simulink model "ExampleAdditionalVehicle"  (Simulink 9.2)
settings: Solver=FixedStepDiscrete  StartTime=0.0  StopTime=inf  FixedStep=0.001  RelTol=1e-3  EnableMultiTasking=on
libraries: rFproPhysicsLib x15, simulink x2
settings Model: Creator=enewton  LastModifiedBy=SeanKavanagh  ParamWorkspaceSource=ReferencedWorkspace  TunableVars=LOCAL_PORT_RECV,REMOTE_PORT_RECV,gCGHeight,gFrontTrack,gFrontWheelRadius,gLeftWheelBase,gRearTrack,gRearWheelRadius,gRightWheelBase  TunableVarsStorageClass=Auto,Auto,Auto,Auto,Auto,Auto,Auto,Auto,Auto  TunableVarsTypeQualifier=,,,,,,,,
settings OptimizationCC: DefaultParameterBehavior=Inlined  ExpressionDepthLimit=2147483647
settings DebuggingCC: SolverPrmCheckMsg=warning
settings HardwareCC: TargetBitPerPointer=64  TargetBitPerSizeT=64  TargetBitPerPtrDiffT=64  TargetLongLongMode=on  TargetIntDivRoundTo=Zero  TargetEndianess=LittleEndian  TargetWordSize=64  TargetHWDeviceType=MATLAB Host  ProdEqTarget=off
settings RTWCC: SystemTargetFile=rfpro.tlc  MakeCommand="make_rtw OPTS=\"-DRUN_PHYSICS\""  TemplateMakefile=rfpro.tmf  Description=rFpro Target (Run Physics)  TargetLang=C++  RTWCompilerOptimization=on
settings STFCustomTargetCC: ModelReferenceCompliant=off  GeneratePreprocessorConditionals=Disable all  CombineOutputUpdateFcns=on  MatFileLogging=on  CPPClassGenCompliant=on  GRTInterface=off  SystemTargetFile=rfpro.tlc
settings GRTTargetCC: ModelReferenceCompliant=off  ParMdlRefBuildCompliant=off  CompOptLevelCompliant=off  ConcurrentExecutionCompliant=off  CombineOutputUpdateFcns=on  GRTInterface=off  UseToolchainInfoCompliant=off

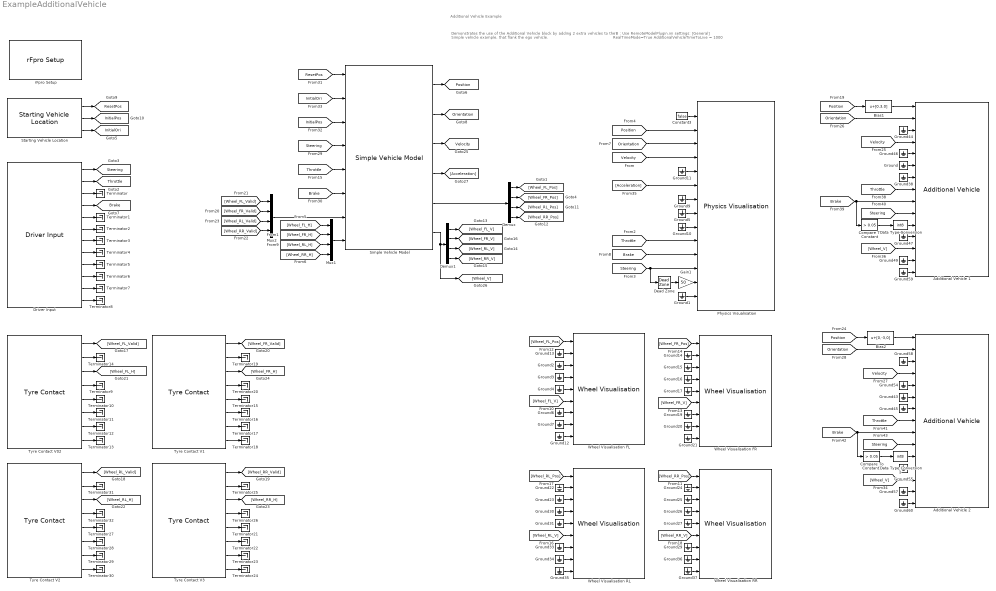
== system ExampleAdditionalVehicle ==
  note: NB : Use RemoteModelPlugin.ini settings:
      |
      | [General]
      | RealTimeMode=True
      | AdditionalVehicleTimeToLive = 1000
  note: Additional Vehicle Example
  note: Demonstrates the use of the Additional Vehicle block
      | by adding 2 extra vehicles to the Simple vehicle example,
      | that flank the ego vehicle.
  Additional Vehicle 1 : rFproPhysicsLib/Additional Vehicle  VEH_FILE='Hatchback_AWD_Red'  DRIVER_NAME=''  UPGRADE_PACK=0  SKIN=''  HELMET=''  COLLIDABLE=off  TRANSPARENT_PROXIMITY=0  MANUAL_TRANSPARENCY=0  HEIGHT_VALID=off  ORI_VALID=on  HEADING_VALID=off  VEL_VALID=on  ROT_VALID=off  GEAR_VALID=off  RPM_VALID=off  INPUTS_VALID=on  BRAKE_LIGHT_VALID=on  HEADLIGHT_VALID=off  WHEEL_ROTATIONS_VALID=on  WHEEL_BRAKE_TEMPS_VALID=off  WHEEL_HEIGHTS_VALID=off  period=0.01  offset=0  useReverseByteOrder=on  rFpro__platform=Remote Model - Default
  Additional Vehicle 2 : rFproPhysicsLib/Additional Vehicle  VEH_FILE='Hatchback_AWD_Red'  DRIVER_NAME=''  UPGRADE_PACK=0  SKIN=''  HELMET=''  COLLIDABLE=off  TRANSPARENT_PROXIMITY=0  MANUAL_TRANSPARENCY=0  HEIGHT_VALID=off  ORI_VALID=on  HEADING_VALID=off  VEL_VALID=on  ROT_VALID=off  GEAR_VALID=off  RPM_VALID=off  INPUTS_VALID=on  BRAKE_LIGHT_VALID=on  HEADLIGHT_VALID=off  WHEEL_ROTATIONS_VALID=on  WHEEL_BRAKE_TEMPS_VALID=off  WHEEL_HEIGHTS_VALID=off  period=0.01  offset=0  useReverseByteOrder=on  rFpro__platform=Remote Model - Default
  Bias1 : Bias  Bias=[0,3,0]
  Bias2 : Bias  Bias=[0,-3,0]
  Compare To Constant : simulink/Logic and Bit Operations/Compare To Constant  relop=>  const=0.05  OutDataTypeStr=uint8
  Compare To Constant1 : simulink/Logic and Bit Operations/Compare To Constant  relop=>  const=0.05  OutDataTypeStr=uint8
  Constant3 : Constant  Value=false
  Data Type Conversion : DataTypeConversion  OutDataTypeStr=int8
  Data Type Conversion1 : DataTypeConversion  OutDataTypeStr=int8
  Dead Zone : DeadZone  LowerValue=-0.05  UpperValue=0.05  SaturateOnIntegerOverflow=on
  Demux : Demux
  Demux1 : Demux
  Driver Input : rFproPhysicsLib/Driver Input
  Gain1 : Gain  Gain=50
  Ground{,1..7,9..17,19..27,29..31,33..38,43..47,49,54..55,57..60} (47 alike) : Ground
  Mux1 : Mux
  Mux2 : Mux
  Physics Visualisation : rFproPhysicsLib/Physics Visualisation  PAR_SKIP_INTERNAL_PHYSICS=off  PAR_ACCEL_VALID=on  PAR_ROT_ACCEL_VALID=off  PAR_GEAR_VALID=off  PAR_RPM_VALID=on  PAR_INPUTS_VALID=on  PAR_STEER_TORQUE_VALID=on  PAR_HEADLIGHTS_ON_VALID=off  PAR_WHEEL_POS_VALID=on  PAR_WHEEL_ORI_VALID=off  PAR_TYRE_PARAMS_VALID=off  PAR_WHEEL_ROTATION_VALID=on  PAR_WHEEL_BRAKE_TEMP_VALID=off  PAR_WHEEL_TREAD_TEMP_VALID=off  PAR_WHEEL_AIR_TEMP_VALID=off  period=-1  offset=0  useReverseByteOrder=on  rFpro__platform=Remote Model - Default
  Simple Vehicle Model : rFproPhysicsLib/Internal Utility/Simple Vehicle Model  TIMESTEP=0.001  gCGHeight=0.5  gLeftWheelBase=2.626  gRightWheelBase=2.626  gFrontTrack=1.55  gRearTrack=1.525  gFrontWheelRadius=0.32  gRearWheelRadius=0.33  gWheelDeflection=0
  Starting Vehicle Location : rFproPhysicsLib/Starting Vehicle Location  cg_offset=CG_OFFSET_FROM_NOSE  numPackets=1  rFpro__platform=Remote Model - Default
  Terminator{,1..32} (33 alike) : Terminator
  Tyre Contact V02 : rFproPhysicsLib/Tyre Contact  LabelModeActiveChoice=rFproLib_RemoteModel  wheel=FL  contact=[]  radius=0.32  width=0.25  sampleTime=-1  rFpro__platform=Remote Model - Default
  Tyre Contact V1 : rFproPhysicsLib/Tyre Contact  LabelModeActiveChoice=rFproLib_RemoteModel  wheel=FR  contact=[]  radius=0.32  width=0.25  sampleTime=-1  rFpro__platform=Remote Model - Default
  Tyre Contact V2 : rFproPhysicsLib/Tyre Contact  LabelModeActiveChoice=rFproLib_RemoteModel  wheel=RL  contact=[]  radius=0.33  width=0.25  sampleTime=-1  rFpro__platform=Remote Model - Default
  Tyre Contact V3 : rFproPhysicsLib/Tyre Contact  LabelModeActiveChoice=rFproLib_RemoteModel  wheel=RR  contact=[]  radius=0.33  width=0.25  sampleTime=-1  rFpro__platform=Remote Model - Default
  Wheel Visualisation FL : rFproPhysicsLib/Wheel Visualisation  wheelStr=FL
  Wheel Visualisation FR : rFproPhysicsLib/Wheel Visualisation  wheelStr=FR
  Wheel Visualisation RL : rFproPhysicsLib/Wheel Visualisation  wheelStr=RL
  Wheel Visualisation RR : rFproPhysicsLib/Wheel Visualisation  wheelStr=RR
  rFpro Setup : rFproPhysicsLib/rFpro Setup  platform=Remote Model - Default  stopOnSessionEnd=on  usePseudoRealtime=on  syncToRF=on  useReverseByteOrder=off  useRfTime=on  minIterations=4  maxIterations=1000  ipReceiveAddress='127.0.0.1'  ipReceivePort=11054  receiveSampleTime=-1  ipTransmitAddress='127.0.0.1'  ipTransmitPort=11052  transmitSampleTime=-1  pluginType=RUN_PHYSICS  sysTarget=xpctarget.tlc  templateMakeFile=xpc_default_tmf  makeCommand=make_rtw  buildDesc=xPC target
  tag scope: Brake=global, InitialOri=global, InitialPos=global, Orientation=global, Position=global, ResetPos=global, Steering=global, Throttle=global, Velocity=global
  wires:
  Starting Vehicle Location/2 -> [InitialPos]
  Constant3/1 -> Physics Visualisation/1
  [Orientation] -> Physics Visualisation/3
  [Velocity] -> Physics Visualisation/4
  [Throttle] -> Physics Visualisation/10
  [Steering] -> Dead Zone/1, Physics Visualisation/12
  [Brake] -> Physics Visualisation/11
  Driver Input/1 -> [Steering]
  Driver Input/2 -> [Throttle]
  Driver Input/4 -> [Brake]
  [Position] -> Physics Visualisation/2
  Driver Input/3 -> Terminator/1
  Driver Input/5 -> Terminator1/1
  Driver Input/6 -> Terminator2/1
  Driver Input/7 -> Terminator3/1
  Driver Input/8 -> Terminator4/1
  Driver Input/9 -> Terminator5/1
  Driver Input/10 -> Terminator6/1
  Driver Input/11 -> Terminator7/1
  Driver Input/12 -> Terminator8/1
  [Acceleration] -> Physics Visualisation/6
  Ground9/1 -> Physics Visualisation/7
  Ground10/1 -> Physics Visualisation/9
  Ground11/1 -> Physics Visualisation/5
  Starting Vehicle Location/1 -> [ResetPos]
  Gain1/1 -> Physics Visualisation/13
  Ground1/1 -> Physics Visualisation/14
  Tyre Contact V02/4 -> Terminator9/1
  Tyre Contact V02/5 -> Terminator10/1
  Tyre Contact V02/6 -> Terminator11/1
  Ground2/1 -> Wheel Visualisation FL/3
  Ground3/1 -> Wheel Visualisation FL/4
  Ground4/1 -> Wheel Visualisation FL/5
  Ground6/1 -> Wheel Visualisation FL/7
  Ground7/1 -> Wheel Visualisation FL/8
  Ground12/1 -> Wheel Visualisation FL/9
  Ground13/1 -> Wheel Visualisation FL/2
  Tyre Contact V02/7 -> Terminator12/1
  Tyre Contact V02/2 -> Terminator14/1
  Tyre Contact V02/8 -> Terminator13/1
  Ground14/1 -> Wheel Visualisation FR/2
  Ground15/1 -> Wheel Visualisation FR/3
  Ground16/1 -> Wheel Visualisation FR/4
  Ground17/1 -> Wheel Visualisation FR/5
  Ground19/1 -> Wheel Visualisation FR/7
  Ground20/1 -> Wheel Visualisation FR/8
  Ground21/1 -> Wheel Visualisation FR/9
  Tyre Contact V1/5 -> Terminator15/1
  Tyre Contact V1/6 -> Terminator16/1
  Tyre Contact V1/2 -> Terminator19/1
  Tyre Contact V1/8 -> Terminator18/1
  Ground22/1 -> Wheel Visualisation RL/2
  Ground23/1 -> Wheel Visualisation RL/3
  Ground30/1 -> Wheel Visualisation RL/4
  Ground31/1 -> Wheel Visualisation RL/5
  Ground33/1 -> Wheel Visualisation RL/7
  Ground34/1 -> Wheel Visualisation RL/8
  Ground35/1 -> Wheel Visualisation RL/9
  Tyre Contact V2/4 -> Terminator32/1
  Tyre Contact V2/5 -> Terminator27/1
  Tyre Contact V2/6 -> Terminator28/1
  Tyre Contact V2/7 -> Terminator29/1
  Tyre Contact V2/2 -> Terminator31/1
  Tyre Contact V2/8 -> Terminator30/1
  Ground24/1 -> Wheel Visualisation RR/2
  Ground25/1 -> Wheel Visualisation RR/3
  Ground26/1 -> Wheel Visualisation RR/4
  Ground27/1 -> Wheel Visualisation RR/5
  Ground29/1 -> Wheel Visualisation RR/7
  Ground36/1 -> Wheel Visualisation RR/8
  Ground37/1 -> Wheel Visualisation RR/9
  Tyre Contact V3/4 -> Terminator26/1
  Tyre Contact V3/5 -> Terminator21/1
  Tyre Contact V3/6 -> Terminator22/1
  Tyre Contact V3/7 -> Terminator23/1
  Tyre Contact V3/2 -> Terminator25/1
  Tyre Contact V3/8 -> Terminator24/1
  [Position] -> Bias1/1
  Bias1/1 -> Additional Vehicle 1/1
  Ground/1 -> Additional Vehicle 1/6
  Ground38/1 -> Additional Vehicle 1/7
  [Throttle] -> Additional Vehicle 1/8
  [Brake] -> Compare To Constant/1, Additional Vehicle 1/9
  [Steering] -> Additional Vehicle 1/10
  [Orientation] -> Additional Vehicle 1/2
  [Velocity] -> Additional Vehicle 1/4
  Ground46/1 -> Additional Vehicle 1/5
  Ground47/1 -> Additional Vehicle 1/12
  [Wheel_V] -> Additional Vehicle 1/13
  Ground49/1 -> Additional Vehicle 1/14
  Ground44/1 -> Additional Vehicle 1/3
  Ground59/1 -> Additional Vehicle 1/15
  Ground5/1 -> Physics Visualisation/8
  [Position] -> Bias2/1
  Bias2/1 -> Additional Vehicle 2/1
  Ground43/1 -> Additional Vehicle 2/6
  Ground45/1 -> Additional Vehicle 2/7
  [Throttle] -> Additional Vehicle 2/8
  [Brake] -> Compare To Constant1/1, Additional Vehicle 2/9
  [Steering] -> Additional Vehicle 2/10
  Ground54/1 -> Additional Vehicle 2/5
  Ground55/1 -> Additional Vehicle 2/12
  [Wheel_V] -> Additional Vehicle 2/13
  Ground57/1 -> Additional Vehicle 2/14
  [Orientation] -> Additional Vehicle 2/2
  [Velocity] -> Additional Vehicle 2/4
  Ground58/1 -> Additional Vehicle 2/3
  Ground60/1 -> Additional Vehicle 2/15
  Simple Vehicle Model/5 -> Demux/1
  Demux/1 -> [Wheel_FL_Pos]
  Demux/2 -> [Wheel_FR_Pos]
  Demux/3 -> [Wheel_RL_Pos]
  Demux/4 -> [Wheel_RR_Pos]
  Demux1/1 -> [Wheel_FL_V]
  Demux1/2 -> [Wheel_FR_V]
  Demux1/3 -> [Wheel_RL_V]
  Demux1/4 -> [Wheel_RR_V]
  Simple Vehicle Model/6 -> [Wheel_V], Demux1/1
  [Wheel_RL_Valid] -> Mux2/3
  [Wheel_RR_Valid] -> Mux2/4
  [Wheel_FL_Valid] -> Mux2/1
  [Wheel_FR_Valid] -> Mux2/2
  [Wheel_FR_H] -> Mux1/2
  [Wheel_FL_H] -> Mux1/1
  [Wheel_RR_H] -> Mux1/4
  [Wheel_RL_H] -> Mux1/3
  Mux2/1 -> Simple Vehicle Model/7
  Mux1/1 -> Simple Vehicle Model/8
  Tyre Contact V1/1 -> [Wheel_FR_Valid]
  Tyre Contact V1/3 -> [Wheel_FR_H]
  Tyre Contact V3/1 -> [Wheel_RR_Valid]
  Tyre Contact V3/3 -> [Wheel_RR_H]
  Tyre Contact V2/1 -> [Wheel_RL_Valid]
  Tyre Contact V2/3 -> [Wheel_RL_H]
  Tyre Contact V02/1 -> [Wheel_FL_Valid]
  Tyre Contact V02/3 -> [Wheel_FL_H]
  [Wheel_FR_Pos] -> Wheel Visualisation FR/1
  [Wheel_FR_V] -> Wheel Visualisation FR/6
  [Wheel_FL_Pos] -> Wheel Visualisation FL/1
  [Wheel_FL_V] -> Wheel Visualisation FL/6
  [Wheel_RR_Pos] -> Wheel Visualisation RR/1
  [Wheel_RR_V] -> Wheel Visualisation RR/6
  [Wheel_RL_V] -> Wheel Visualisation RL/6
  [Wheel_RL_Pos] -> Wheel Visualisation RL/1
  Starting Vehicle Location/3 -> [InitialOri]
  [Steering] -> Simple Vehicle Model/4
  [Throttle] -> Simple Vehicle Model/5
  [Brake] -> Simple Vehicle Model/6
  [ResetPos] -> Simple Vehicle Model/1
  [InitialPos] -> Simple Vehicle Model/3
  [InitialOri] -> Simple Vehicle Model/2
  Simple Vehicle Model/1 -> [Position]
  Simple Vehicle Model/2 -> [Orientation]
  Simple Vehicle Model/3 -> [Velocity]
  Tyre Contact V1/4 -> Terminator20/1
  Tyre Contact V1/7 -> Terminator17/1
  Simple Vehicle Model/4 -> [Acceleration]
  Dead Zone/1 -> Gain1/1
  Compare To Constant/1 -> Data Type Conversion/1
  Compare To Constant1/1 -> Data Type Conversion1/1
  Data Type Conversion/1 -> Additional Vehicle 1/11
  Data Type Conversion1/1 -> Additional Vehicle 2/11
